simulink model "examples_of_saturation_block"  (R2021a)
settings: Solver=VariableStepAuto  StartTime=0.0  StopTime=10  MaxStep=1e-3  RelTol=1e-3
libraries: simulink x1
settings Model: Creator=YasserNet  LastModifiedBy=YasserNet

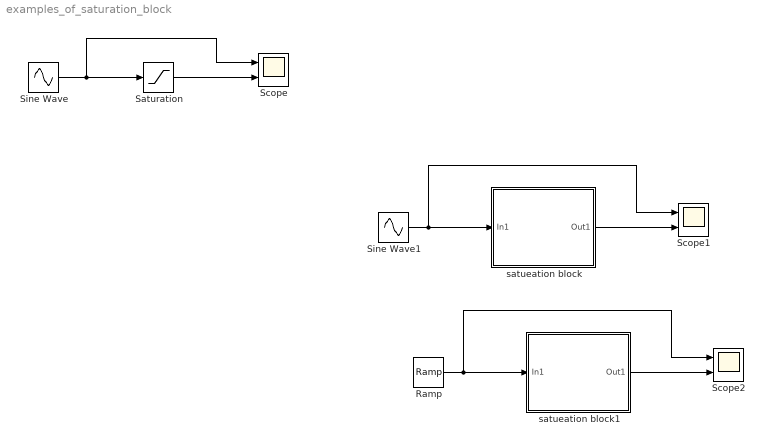
== system examples_of_saturation_block ==
  Ramp : simulink/Sources/Ramp  slope=1  start=3  InitialOutput=8
  Saturation : Saturate
  Scope : Scope  NumInputPorts=2
  Scope1 : Scope  NumInputPorts=2
  Scope2 : Scope  NumInputPorts=2
  Sine Wave : Sin  Amplitude=5  Frequency=2*2*pi  SampleTime=0
  Sine Wave1 : Sin  Amplitude=5  Frequency=2*2*pi  SampleTime=0
  satueation block : Subsystem
  satueation block1 : Subsystem
  wires:
  Saturation/1 -> Scope/2
  Sine Wave/1 -> Scope/1, Saturation/1
  Sine Wave1/1 -> Scope1/1, satueation block/1(In1)
  satueation block/1(Out1) -> Scope1/2
  satueation block1/1(Out1) -> Scope2/2
  Ramp/1 -> satueation block1/1(In1), Scope2/1

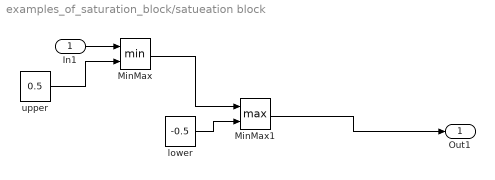
== system examples_of_saturation_block/satueation block ==
  In1 : Inport
  MinMax : MinMax  Inputs=2
  MinMax1 : MinMax  Function=max  Inputs=2
  lower : Constant  Value=-0.5
  upper : Constant  Value=0.5
  Out1 : Outport
  wires:
  upper/1 -> MinMax/2
  MinMax/1 -> MinMax1/1
  MinMax1/1 -> Out1/1
  lower/1 -> MinMax1/2
  In1/1 -> MinMax/1

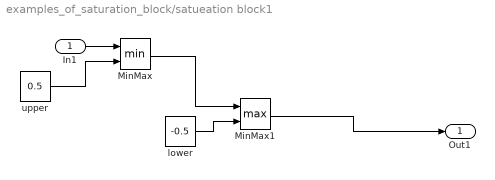
== system examples_of_saturation_block/satueation block1 ==
  In1 : Inport
  MinMax : MinMax  Inputs=2
  MinMax1 : MinMax  Function=max  Inputs=2
  lower : Constant  Value=-0.5
  upper : Constant  Value=0.5
  Out1 : Outport
  wires:
  In1/1 -> MinMax/1
  lower/1 -> MinMax1/2
  MinMax1/1 -> Out1/1
  MinMax/1 -> MinMax1/1
  upper/1 -> MinMax/2
